simulink model "pinv_model"  (R2018b)
settings: Solver=VariableStepAuto  StartTime=0.0  StopTime=300  RelTol=1e-3
values from neighbouring files (symbols this model uses):
  heave_data =     [heave_data.mat]
  pseudoSS =     [pseudoSS.mat]
  surge_data =     [surge_data.mat]
undefined symbols (not defined in the file or in its folder): seaWave, SS_full
settings Model: Creator=user  LastModifiedBy=user

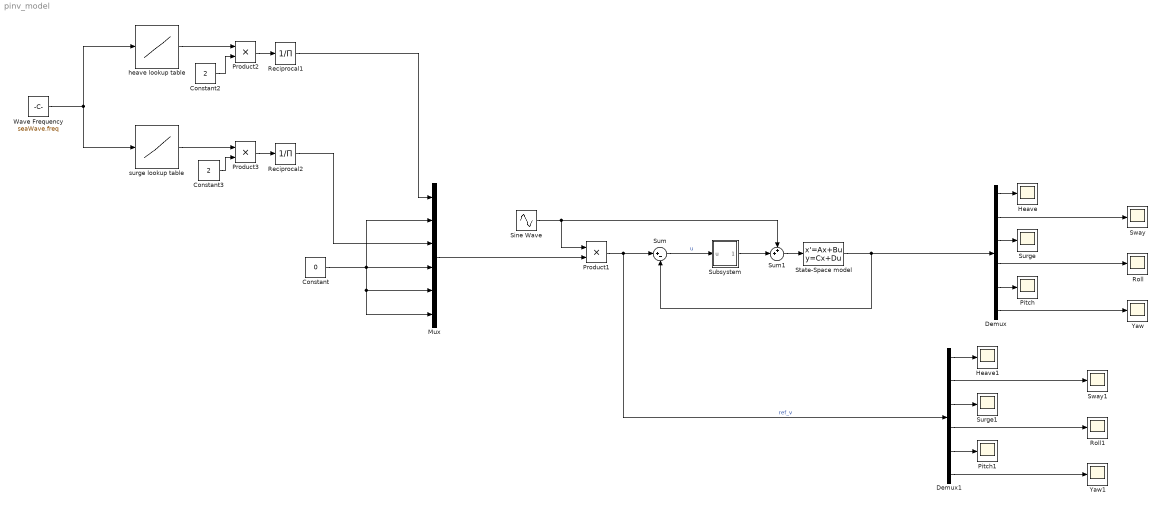
== system pinv_model ==
  Constant : Constant  Value=0
  Constant2 : Constant  Value=2
  Constant3 : Constant  Value=2
  Demux : Demux  Outputs=6
  Demux1 : Demux  Outputs=6
  Heave : Scope
  Heave1 : Scope
  Mux : Mux  Inputs=6
  Pitch : Scope
  Pitch1 : Scope
  Product1 : Product
  Product2 : Product
  Product3 : Product
  Reciprocal1 : Product  Inputs=/
  Reciprocal2 : Product  Inputs=/
  Roll : Scope
  Roll1 : Scope
  Sine Wave : Sin  Amplitude=seaWave.amp  Frequency=seaWave.freq  SampleTime=0
  State-Space model : StateSpace  A=SS_full.A  B=SS_full.B  C=SS_full.C  D=SS_full.D  InitialCondition=0
  Subsystem : Subsystem
      mask Display: fprintf("K")
  Sum : Sum  Inputs=|+-
  Sum1 : Sum  Inputs=++|
  Surge : Scope
  Surge1 : Scope
  Sway : Scope
  Sway1 : Scope
  Wave Frequency : Constant  Value=seaWave.freq
  Yaw : Scope
  Yaw1 : Scope
  heave lookup table : Lookup_n-D  NumberOfTableDimensions=1  BreakpointsForDimension1=heave_data.freq  Table=heave_data.amplitudes  InternalRulePriority=Speed  RndMeth=Simplest  InputSameDT=on
  surge lookup table : Lookup_n-D  NumberOfTableDimensions=1  BreakpointsForDimension1=surge_data.freq  Table=surge_data.amplitudes  InternalRulePriority=Speed  RndMeth=Simplest  InputSameDT=on
  wires:
  Wave Frequency/1 -> surge lookup table/1, heave lookup table/1
  Constant/1 -> Mux/5, Mux/6, Mux/2, Mux/4
  Mux/1 -> Product1/2
  Product1/1 -> Demux1/1, Sum/1  "ref_v"
  Sine Wave/1 -> Sum1/1, Product1/1
  Demux/1 -> Heave/1
  Demux/3 -> Surge/1
  Demux/5 -> Pitch/1
  Sum1/1 -> State-Space model/1
  Sum/1 -> Subsystem/1(u)  "u"
  Subsystem/1(Out2) -> Sum1/2
  Demux/2 -> Sway/1
  Demux/4 -> Roll/1
  Demux/6 -> Yaw/1
  heave lookup table/1 -> Product2/1
  Constant2/1 -> Product2/2
  Product2/1 -> Reciprocal1/1
  Reciprocal1/1 -> Mux/1
  surge lookup table/1 -> Product3/1
  Constant3/1 -> Product3/2
  Product3/1 -> Reciprocal2/1
  Reciprocal2/1 -> Mux/3
  Demux1/6 -> Yaw1/1
  Demux1/5 -> Pitch1/1
  Demux1/2 -> Sway1/1
  Demux1/4 -> Roll1/1
  Demux1/3 -> Surge1/1
  Demux1/1 -> Heave1/1
  State-Space model/1 -> Demux/1, Sum/2

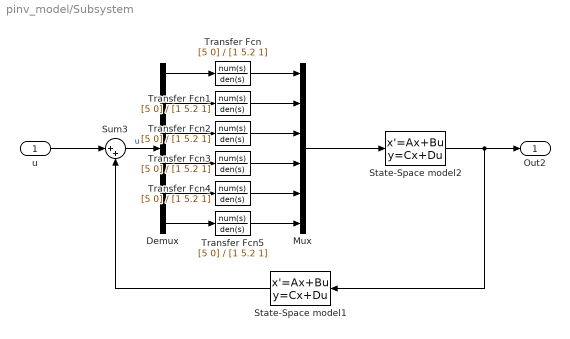
== system pinv_model/Subsystem ==
  u : Inport
  Demux : Demux  Outputs=6
  Mux : Mux  Inputs=6
  State-Space model1 : StateSpace  A=SS_full.A  B=SS_full.B  C=SS_full.C  D=SS_full.D  InitialCondition=0
  State-Space model2 : StateSpace  A=pseudoSS.A  B=pseudoSS.B  C=pseudoSS.C  D=pseudoSS.D  InitialCondition=0
  Sum3 : Sum  Inputs=|++
  Transfer Fcn{,1..5} (6 alike) : TransferFcn  Numerator=[5 0]  Denominator=[1 5.2 1]
  Out2 : Outport
  wires:
  Sum3/1 -> Demux/1  "u"
  Demux/1 -> Transfer Fcn/1
  State-Space model1/1 -> Sum3/2
  u/1 -> Sum3/1
  Demux/2 -> Transfer Fcn1/1
  Demux/3 -> Transfer Fcn2/1
  Demux/4 -> Transfer Fcn3/1
  Demux/5 -> Transfer Fcn4/1
  Demux/6 -> Transfer Fcn5/1
  Transfer Fcn/1 -> Mux/1
  Transfer Fcn1/1 -> Mux/2
  Transfer Fcn2/1 -> Mux/3
  Transfer Fcn3/1 -> Mux/4
  Transfer Fcn4/1 -> Mux/5
  Transfer Fcn5/1 -> Mux/6
  Mux/1 -> State-Space model2/1
  State-Space model2/1 -> State-Space model1/1, Out2/1
